simulink library "Lib_SENSOR"  (R2016a)
settings: Solver=ode45  StartTime=0.0  StopTime=10.0  RelTol=1e-3
settings Model: Creator=michaelstolz  LastModifiedBy=meh97
settings DataIOCC: LimitDataPoints=on  SaveFormat=Array  SignalLoggingSaveFormat=ModelDataLogs
settings OptimizationCC: ExpressionDepthLimit=2147483647
settings DebuggingCC: UnderspecifiedInitializationDetection=Classic  MergeDetectMultiDrivingBlocksExec=none  SolverPrmCheckMsg=warning  FcnCallInpInsideContextMsg=EnableAllAsWarning  StateNameClashWarn=warning
settings HardwareCC: ProdBitPerPointer=32  ProdLargestAtomicFloat=None  ProdIntDivRoundTo=Undefined  ProdEndianess=Unspecified  ProdWordSize=32  ProdHWDeviceType=32-bit Generic
settings ModelReferenceCC: PropagateSignalLabelsOutOfModel=off

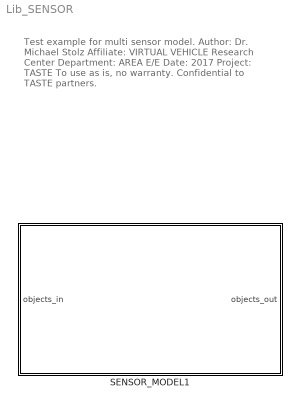
== system Lib_SENSOR ==
  note: Test example for multi sensor model.
      | Author: Dr. Michael Stolz
      | Affiliate: VIRTUAL VEHICLE Research Center
      | Department: AREA E/E
      | Date: 2017
      | Project: TASTE
      | To use as is, no warranty.
      | Confidential to TASTE partners.
  SENSOR_MODEL1 : Subsystem  mask(SENSOR MODELS){NumObjects_=150, MountX_=[0,-4], MountY_=[0,0], MountA_=[0,180], SensorModel_=RBF Model, SensorAngle_=[20,60], SensorRange_=[80,40], SensorXY_={ [0   11  25  40 55  70  85 95 100;  0   7  12  16 19 20  19 10 0 ], [0   6.5  12.5  20 27.5  35  42.5 47.5 41;  0   7  12  16 19 20  19 10 0 ] }, SensorVisibility_=Cascaded case selection, SensorSegmentation_=5, SensorMinVis_=50, SensorType_={'R','C'}, NrSensors_=1}
      mask prompts: NumObjects_ "Object Bus Dimension"; MountX_ "Mounting location x direction"; MountY_ "Mountnig location y direction [m]"; MountA_ "Mounting Orientation [°]"; SensorModel_ "Sensor Model"; SensorAngle_ "Sensor Angle [°]"; SensorRange_ "Sensor Range [m]"; SensorXY_ "Sensor Configuration { [ n x 2] , [m x 2], ... }"; SensorVisibility_ "Visibility Algorithm"; SensorSegmentation_ "Segmentation Number [-]"; SensorMinVis_ "Minimum Visibility [%]"; SensorType_ "Sensor Type {'R', 'L', 'C', ... }"; NrSensors_ "Number of Sensors"
      mask help:
      | First configurate the size of the incoming bus by telling how many objects
      | are used (a fixed value).
      | Then enter the sensor model parameters.
      | The sensor models can be either sector of RBF models.
      | For visibility detection you can select on of two different approaches.
      |
      | (C) VIRTUAL VEHICLE Research Center 2017
      | within TASTE Project
      | Author Dr. Michael Stolz (michael.stolz@v2c2.at)
      |
      | This software is development software used for research.
      | Although checked intensively, use at own risk.
      mask Help:
      | See the documentation in the code or the documentation of the TASTE
      | FFG-Project.
      mask TypeOptions NumObjects_: SENSOR_MODEL_SF/NumObjects
      mask Callback NumObjects_:
      | if isempty(get_param(gcb,'NumObjects_')),
      |     set_param(gcb, 'NumObjects_','3');
      | end
      mask TypeOptions MountX_: SENSOR_MODEL_SF/MountX
      mask Callback MountX_:
      | if isempty(get_param(gcb,'MountX_')),
      |     set_param(gcb, 'MountX_','[0,-4]');
      | end
      mask TypeOptions MountY_: SENSOR_MODEL_SF/MountY
      mask Callback MountY_:
      | if isempty(get_param(gcb,'MountY_')),
      |     set_param(gcb, 'MountY_','[0,0]');
      | end
      mask TypeOptions MountA_: SENSOR_MODEL_SF/MountA
      mask Callback MountA_:
      | if isempty(get_param(gcb,'MountA_')),
      |     set_param(gcb, 'MountA_','[0,-180]');
      | end
      mask TypeOptions SensorModel_: SENSOR_MODEL_SF/SensorModel
      mask Callback SensorModel_:
      | e123344tmp = get_param(gcb,'MaskEnables');
      | 
      | switch get_param(gcb,'SensorModel_'),
      |     case 'Sector Model',
      |         e123344tmp{find(strcmp(get_param(gcb,'MaskNames'),'SensorRange_'))} = 'on';
      |         e123344tmp{find(strcmp(get_param(gcb,'MaskNames'),'SensorAngle_'))} = 'on';
      |         e123344tmp{find(strcmp(get_param(gcb,'MaskNames'),'SensorXY_'))} = 'off';
      |     case 'RBF Model',
      |         e123344tmp{find(strcmp(get_param(gcb,'MaskNames'),'SensorRange_'))} = 'off';
      |         e123344tmp{find(strcmp(get_param(gcb,'MaskNames'),'SensorAngle_'))} = 'off';
      |         e123344tmp{find(strcmp(get_param(gcb,'MaskNames'),'SensorXY_'))} = 'on';
      |     otherwise,
      |         ;
      | end
      | set_param(gcb,'MaskEnables',e123344tmp);
      | clear e123344tmp
      mask TypeOptions SensorAngle_: SENSOR_MODEL_SF/SensorAngle
      mask Callback SensorAngle_:
      | if isempty(get_param(gcb,'SensorAngle_')),
      |     set_param(gcb, 'SensorAngle_','[60,60]');
      | end
      mask TypeOptions SensorRange_: SENSOR_MODEL_SF/SensorRange
      mask Callback SensorRange_:
      | if isempty(get_param(gcb,'SensorRange_')),
      |     set_param(gcb, 'SensorRange_','[100,60]');
      | end
      mask TypeOptions SensorXY_: SENSOR_MODEL_SF/SensorXY
      mask TypeOptions SensorVisibility_: SENSOR_MODEL_SF/SensorVisibility
      mask Callback SensorVisibility_:
      | e123344tmp = get_param(gcb,'MaskEnables');
      | 
      | 
      | switch get_param(gcb,'SensorVisibility_'),
      |     case 'Cascaded case selection',
      |         e123344tmp{find(strcmp(get_param(gcb,'MaskNames'),'SensorSegmentation_'))} = 'off';
      |     case 'Segmentation',
      |         e123344tmp{find(strcmp(get_param(gcb,'MaskNames'),'SensorSegmentation_'))} = 'on';
      |     otherwise,
      |         ;
      | end
      | set_param(gcb,'MaskEnables',e123344tmp);
      | clear e123344tmp
      mask TypeOptions SensorSegmentation_: SENSOR_MODEL_SF/SensorSegmentation
      mask Callback SensorSegmentation_:
      | if isempty(get_param(gcb,'SensorSegmentation_')),
      |     set_param(gcb, 'SensorSegmentation_','10');
      | end
      mask TypeOptions SensorMinVis_: SENSOR_MODEL_SF/SensorMinVis
      mask Callback SensorMinVis_:
      | if isempty(get_param(gcb,'SensorMinVis_')),
      |     set_param(gcb, 'SensorMinVis_','10');
      | end
      mask TypeOptions SensorType_: SENSOR_MODEL_SF/SensorType
      mask Callback SensorType_:
      | if isempty(get_param(gcb,'SensorType_')),
      |     set_param(gcb, 'SensorType_','{''C'';''R''}');
      | end
      mask TypeOptions NrSensors_: SENSOR_MODEL_SF/NrSensors
      mask Display:
      | text(.5,.7,'\fontname{palatino}\fontsize{15}\bf Sensor Model',...
      |       'HorizontalAlignment','center','texmode','on');
      | text(.5,.3,sprintf('OBJECT BUS DIMENSION: %d',NumObjects_),...
      |       'HorizontalAlignment','center','texmode','off');
      | 
      | port_label('input',1,'objects bus');
      | port_label('output',1,'objects bus');

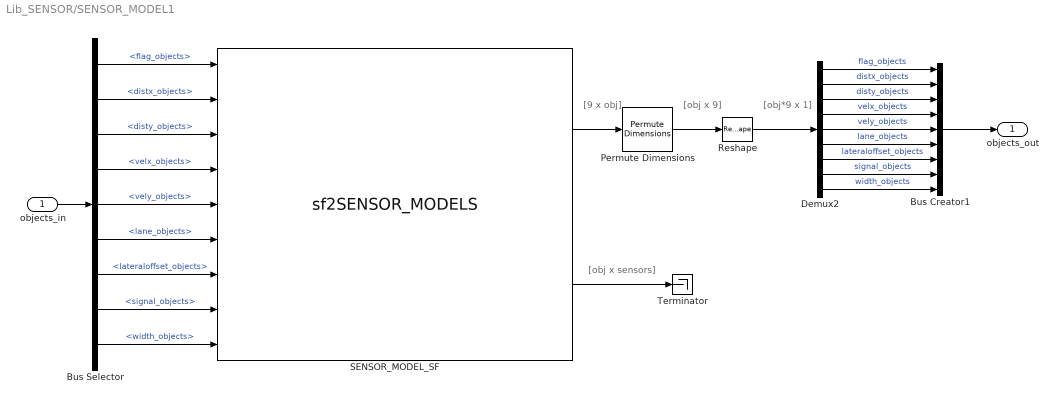
== system Lib_SENSOR/SENSOR_MODEL1 ==
  note: [obj x sensors]
  note: [obj*9 x 1]
  note: [obj x 9]
  note: [9 x obj]
  objects_in : Inport
  Bus Creator1 : BusCreator  Inputs=9
  Bus Selector : BusSelector  OutputSignals=flag_objects,distx_objects,disty_objects,velx_objects,vely_objects,lane_objects,lateraloffset_objects,signal_objects,width_objects
  Demux2 : Demux  Outputs=[-1,-1,-1,-1,-1,-1,-1,-1,-1]
  Permute Dimensions : PermuteDimensions
  Reshape : Reshape
  SENSOR_MODEL_SF : M-S-Function  FunctionName=sf2SENSOR_MODELS  Parameters=NumObjects,MountX,MountY,MountA,SensorModel,SensorRange,SensorXY,SensorVisibility,SensorSegmentation,SensorMinVis,SensorType,SensorAngle  mask(SUMO Simulink Syncronisation){NumObjects=NumObjects_, MountX=MountX_, MountY=MountY_, MountA=MountA_, SensorModel=RBF Model, SensorAngle=SensorAngle_, SensorRange=SensorRange_, SensorXY=SensorXY_, SensorVisibility=Cascaded case selection, SensorSegmentation=SensorSegmentation_, SensorMinVis=SensorMinVis_, SensorType=SensorType_, NrSensors=1}
      mask prompts: NumObjects "Dimension of objects bus"; MountX "Mounting location x direction [m]"; MountY "Mounting location y direction [m]"; MountA "Mounting Orientation [°]"; SensorModel "Sensor Model"; SensorAngle "Sensor Angle [°]"; SensorRange "Sensor Range [m]"; SensorXY "Sensor Configuration { [n x 2], [m x 2] }"; SensorVisibility "Visibility Algorithm"; SensorSegmentation "Segmentation Number [-]"; SensorMinVis "Minimum Visibility [%]"; SensorType "Sensor Type {'R', 'L', 'C', ...}"; NrSensors "Number of Sensors"
      mask TypeOptions SensorModel: Sector Model | RBF Model
      mask TypeOptions SensorVisibility: Cascaded case selection | Segmentation
      mask Display:
      | text(.5,.7,'\fontname{palatino}\fontsize{15}\bf Sensor Model sFunction',...
      |       'HorizontalAlignment','center','texmode','on');
      | text(.5,.4,sprintf('OBJECT BUS DIMENSION: %d',NumObjects),...
      |       'HorizontalAlignment','center','texmode','off');
      | 
      | port_label('input',1,'flag_objects');
      | port_label('input',2,'distx_objects');
      | port_label('input',3,'disty_objects');
      | port_label('input',4,'velx_objects');
      | port_label('input',5,'vely_objects');
      | port_label('input',6,'lane_objects');
      | port_label('input',7,'lateraloffset_objects');
      | port_label('input',8,'signal_objects');
      | port_label('input',9,'width_objects');
      | port_label('output',1,'objects matrix');
      | port_label('output',2,'objects/sensors detection matrix');
  Terminator : Terminator
  objects_out : Outport
  wires:
  SENSOR_MODEL_SF/2 -> Terminator/1
  Bus Selector/9 -> SENSOR_MODEL_SF/9  "<width_objects>"
  Demux2/9 -> Bus Creator1/9  "width_objects"
  SENSOR_MODEL_SF/1 -> Permute Dimensions/1
  objects_in/1 -> Bus Selector/1
  Bus Selector/8 -> SENSOR_MODEL_SF/8  "<signal_objects>"
  Bus Selector/7 -> SENSOR_MODEL_SF/7  "<lateraloffset_objects>"
  Bus Selector/6 -> SENSOR_MODEL_SF/6  "<lane_objects>"
  Bus Selector/5 -> SENSOR_MODEL_SF/5  "<vely_objects>"
  Bus Selector/4 -> SENSOR_MODEL_SF/4  "<velx_objects>"
  Bus Selector/3 -> SENSOR_MODEL_SF/3  "<disty_objects>"
  Bus Selector/2 -> SENSOR_MODEL_SF/2  "<distx_objects>"
  Bus Selector/1 -> SENSOR_MODEL_SF/1  "<flag_objects>"
  Demux2/1 -> Bus Creator1/1  "flag_objects"
  Demux2/2 -> Bus Creator1/2  "distx_objects"
  Demux2/3 -> Bus Creator1/3  "disty_objects"
  Demux2/4 -> Bus Creator1/4  "velx_objects"
  Demux2/5 -> Bus Creator1/5  "vely_objects"
  Demux2/6 -> Bus Creator1/6  "lane_objects"
  Demux2/7 -> Bus Creator1/7  "lateraloffset_objects"
  Demux2/8 -> Bus Creator1/8  "signal_objects"
  Reshape/1 -> Demux2/1
  Permute Dimensions/1 -> Reshape/1
  Bus Creator1/1 -> objects_out/1
